simulink model "sys1"  (Simulink 7.7)
settings: Solver=ode45  StartTime=0.0  StopTime=5  RelTol=1e-3
values from neighbouring files (symbols this model uses):
  c1_den = conv([a3 1],[a4 1])    [case1.m]
  c1_num = conv([a1 1], [a2 1])    [case1.m]
  input = step_in    (= 1)    [main.m]
  k1 = .03    (= 0.03)    [case1.m]
  p_den = conv([1 1 0], [0.1 1])    [main.m]
  p_num = 100    [main.m]
libraries: simulink x1
settings Model: Creator=Edward  LastModifiedBy=Edward

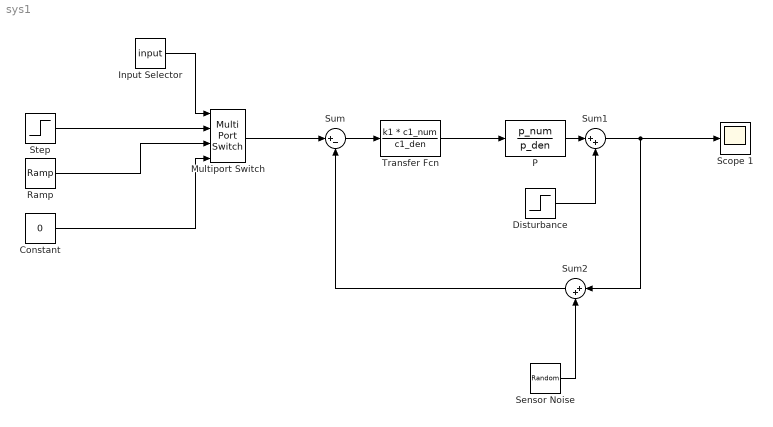
== system sys1 ==
  Constant : Constant  Value=0
  Disturbance : Step  After=0  SampleTime=0
  Input Selector : Constant  Value=input
  Multiport Switch : MultiPortSwitch  zeroidx=off
  P : TransferFcn  Numerator=p_num  Denominator=p_den
  Ramp : simulink/Sources/Ramp  SystemSampleTime=-1  slope=1  start=0  X0=0
  Scope 1 : Scope
  Sensor Noise : RandomNumber  Variance=.1  SampleTime=0.01
  Step : Step  Time=0  SampleTime=0
  Sum : Sum  Inputs=|+-
  Sum1 : Sum  Inputs=|++
  Sum2 : Sum  Inputs=|++
  Transfer Fcn : TransferFcn  Numerator=k1 * c1_num  Denominator=c1_den
  wires:
  P/1 -> Sum1/1
  Sum2/1 -> Sum/2
  Sum1/1 -> Scope 1/1, Sum2/1
  Sensor Noise/1 -> Sum2/2
  Disturbance/1 -> Sum1/2
  Transfer Fcn/1 -> P/1
  Sum/1 -> Transfer Fcn/1
  Step/1 -> Multiport Switch/2
  Multiport Switch/1 -> Sum/1
  Ramp/1 -> Multiport Switch/3
  Input Selector/1 -> Multiport Switch/1
  Constant/1 -> Multiport Switch/4
